simulink model "gpucoder_sobelEdge"  (R2017b)
settings: Solver=VariableStepAuto  StartTime=0.0  StopTime=10  RelTol=1e-3
InitFcn:
  | Isize = single(zeros(240, 320));
  | cfg = coder.gpuConfig('dll');
  | codegen -args {Isize} -config cfg sobelEdge
undefined symbols (not defined in the file or in its folder): gray
libraries: visiongeotforms x1, dspvision x1
CloseFcn:
  | clear Isize cfg;
settings Model: Creator=gvenkata  LastModifiedBy=vravicha

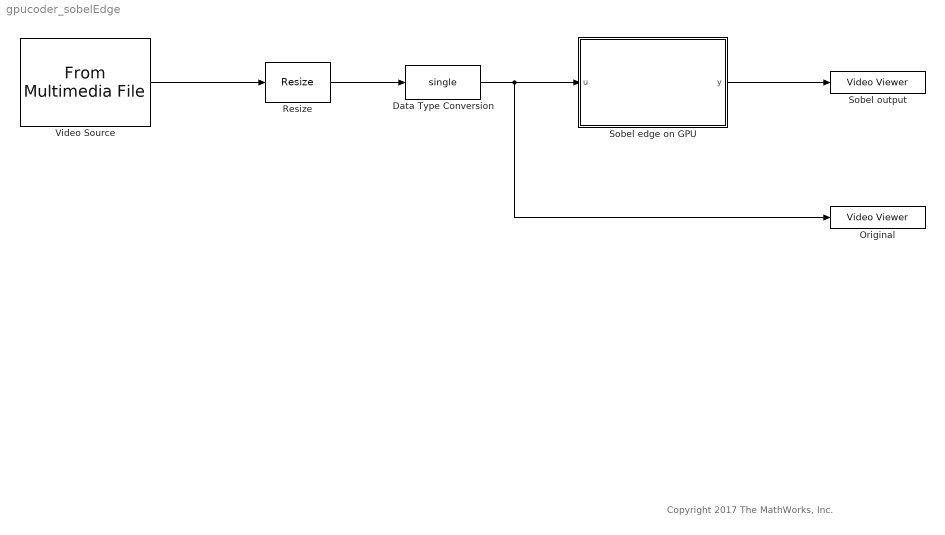
== system gpucoder_sobelEdge ==
  note: Copyright 2017 The MathWorks, Inc.
  Data Type Conversion : DataTypeConversion  OutDataTypeStr=single
  Original : VideoViewer  colormapValue=gray(256)  FigPos=[226 671 467 308]
  Resize : visiongeotforms/Resize  specify=Number of output rows and columns  rfactor=[200 150]  outCols=25  outRows=25  outRowsCols=[size(Isize, 1), size(Isize, 2)]  interp_method=Bilinear  antialias=on  useROI=off  roiFlag=off  prodOutputMode=Binary point scaling  prodOutputWordLength=32  prodOutputFracLength=10  roundingMode=Nearest  overflowMode=on
      settings: SourceProductName=Computer Vision System Toolbox  SourceProductBaseCode=VP
  Sobel edge on GPU : MATLAB Function  TreatAsAtomicUnit=on
  Sobel output : VideoViewer  colormapValue=gray(256)  FigPos=[694 673 456 308]
  Video Source : dspvision/From Multimedia File  inputFilename=visiontraffic.avi  loop=on  numPlays=inf  outputStreams=Video only  videoDataType=double  audioDataType=int16  inheritSampleTime=on  userDefinedSampleTime=402*324  noAudioOutput=off  isIntensityVideo=off  fourcc=Intensity  colorVideoFormat=One multidimensional signal  outputEOF=off  dataOrg=Column-major  audioFrameSize=1024  computeAudioFrameSize=off  outSamplingMode=Sample based
      settings: SourceProductBaseCode=VP
  wires:
  Sobel edge on GPU/1(y) -> Sobel output/1
  Video Source/1 -> Resize/1
  Resize/1 -> Data Type Conversion/1
  Data Type Conversion/1 -> Original/1, Sobel edge on GPU/1(u)

== matlab function gpucoder_sobelEdge/Sobel edge on GPU ==
  data: u input; y output
function y = fcn(u)

y = SobelAPI.sobelEdge(u);

end
